simulink model "weightlose1"  (R2021b)
settings: Solver=VariableStepAuto  StartTime=0.0  StopTime=3000  RelTol=1e-3
libraries: cstblocks x1
settings Model: Creator=DELL  LastModifiedBy=DELL

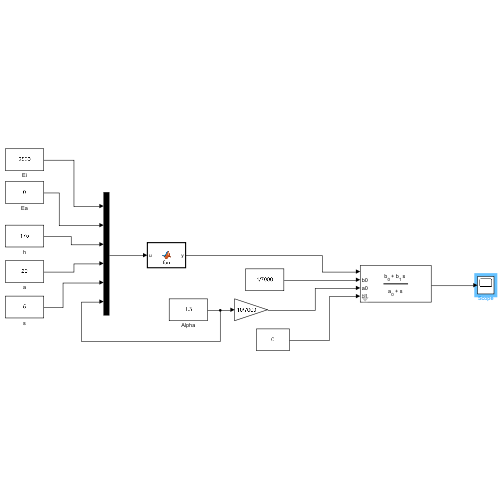
[thumbnail: Simulink's stored preview of the top-level diagram]
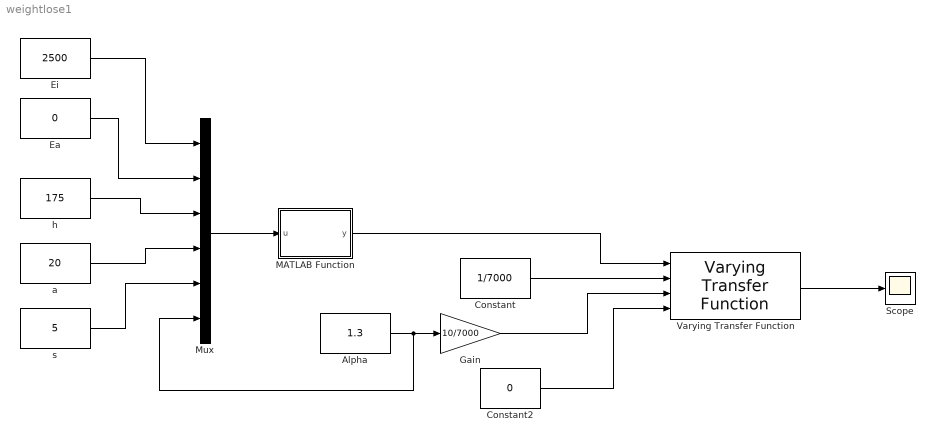
== system weightlose1 ==
  Alpha : Constant  Value=1.3
  Constant : Constant  Value=1/7000
  Constant2 : Constant  Value=0
  Ea : Constant  Value=0
  Ei : Constant  Value=2500
  Gain : Gain  Gain=10/7000
  MATLAB Function : MATLAB Function  TreatAsAtomicUnit=on
  Mux : Mux  Inputs=6
  Scope : Scope
  Varying Transfer Function : cstblocks/Linear Parameter Varying/Varying Transfer Function  N=1
      link override Integrator1: InitialCondition=70
  a : Constant  Value=20
  h : Constant  Value=175
  s : Constant  Value=5
  wires:
  Constant/1 -> Varying Transfer Function/2
  Alpha/1 -> Mux/6, Gain/1
  Gain/1 -> Varying Transfer Function/3
  Constant2/1 -> Varying Transfer Function/4
  Mux/1 -> MATLAB Function/1(u)
  Ei/1 -> Mux/1
  Ea/1 -> Mux/2
  h/1 -> Mux/3
  a/1 -> Mux/4
  s/1 -> Mux/5
  MATLAB Function/1(y) -> Varying Transfer Function/1
  Varying Transfer Function/1 -> Scope/1

== matlab function weightlose1/MATLAB Function ==
  data: u input; y output
function y = fcn(u)

y = u(1)-u(2)-u(6)*(6.25*u(3)-5*u(4)+u(5));
